simulink model "EnablePort2"  (R2017b)
settings: Solver=FixedStepDiscrete  StartTime=0.0  StopTime=10.0  FixedStep=0.200000  RelTol=1e-3
model workspace (MAT data in the model file):
  input_struct.time = [0; 0.2; 0.4; 0.6; 0.8; 1; 1.2; 1.4; 1.6; 1.8; 2; 2.2; 2.4; 2.6; 2.8; 3; 3.2; 3.4; 3.6; 3.8; 4; 4.2; 4.4; 4.6; 4.8; 5; 5.2; 5.4; 5.6; 5.8; 6; 6.2; 6.4; 6.6; 6.8; 7; 7.2; 7.4; 7.6; 7.8; 8; 8.2; 8.4; 8.6; 8.8; 9; 9.2; 9.4; 9.6; 9.8; 10; 10.2; 10.4; 10.6; 10.8; 11; 11.2; 11.4; 11.6; 11.8; 12; 12.2; 12.4; 12.6; 12.8; 13; 13.2; 13.4; 13.6; 13.8; 14; 14.2; 14.4; 14.6; 14.8; 15; 15.2; 15.4; 15.6; 15.8; 16; 16.2; 16.4; 16.6; 16.8; 17; 17.2; 17.4; 17.6; 17.8; 18; 18.2; 18.4; 18.6; 18.8; 19; 19.2; 19.4; 19.6; 19.8]
  input_struct.signals(1).name = 'In1'
  input_struct.signals(1).values = [57.969273693; 82.7041231105; 6.65087199712; 60.8152888981; 12.5320713222; 50.1752903924; -98.1539291241; -4.64302962846; -49.9340946949; -38.4163483162; 93.3898208851; -58.2391278811; 4.09525055477; -54.8907741205; 13.4395747662; 99.6327052148; -73.6269326538; 90.9353169806; -75.2244977004; -62.7523588484; 29.3005421166; -74.3661845002; -83.7358994286; 31.8454108442; -94.5202297837; 97.0359601658; 7.86618942535; -25.2330166582; 41.3469772282; 89.4822748814; -23.5445302312; 38.5817109897; 20.4142624802; 55.0515424276; 18.3668411358; -24.7640384704; 70.1298399192; -54.8529618431; 59.3916568652; 99.3762012577; -43.7378359258; 42.0761950049; 32.9284134306; -17.0328933637; -0.346019545145; 89.8246051015; 90.63633518; 46.5846623372; -23.0639990752; -91.983454233; 16.5867171862; 12.9425283429; -28.9634765103; 76.0401642003; 24.906026599; 24.803109268; -40.8517177427; -85.0640146214; -41.2588011215; -53.052038291; -30.8205238166; 69.6980718111; -67.927123626; -68.427124744; 1.73185392845; 20.6602000119; -67.7206063001; 27.0908649699; 68.7881151707; 56.4538423892; -47.0867291292; -37.0602075398; -63.3608856957; -10.5053454909; -34.6642766771; -44.0367420079; 86.3527816834; -20.0615174075; -24.1153686312; 18.5692898981; -86.2986628105; -58.9524675794; 44.7236556204; 15.0295225661; -59.9534992726; 68.6960690554; -15.2539997979; 8.95019251945; 5.5934767678; -62.978435841; -83.6620572023; -7.18127540382; -93.8890448599; -13.0031684902; 11.5729922646; 27.7564258613; -93.1565173415; 41.9800894582; -66.1352103091; 18.6764946421]
  input_struct.signals(1).dimensions = 1
  input_struct.signals(2).name = 'Enable'
  input_struct.signals(2).values = [21.6129838653; 54.4719173974; -88.7452768515; 70.9450293897; -23.1431348911; -20.0762077942; -34.9165029203; 11.0780220972; -40.9159793561; -26.7759995931; -30.1903342657; 26.0448111076; 32.8884161614; 98.4192673234; 88.8722524324; -29.9304276267; -61.4004110247; 83.9152276745; -42.2615899335; 10.1718855023; 83.8648307629; -81.9902955723; -48.4607395594; -14.5904084585; 15.5446580081; 79.9042789778; -56.3548766014; 93.4063768947; -13.2037243931; 56.9644846349; 5.0467689241; -33.7446294351; -13.6812706476; 43.5803202039; 83.2424156234; 78.0055974736; -73.0587883246; -76.0174489205; 78.6904842168; 30.6171083505; -91.9443846645; 0.943192710913; 78.8906930826; -22.8543071113; -41.5896244284; -53.1926860055; -59.8103285268; -23.9387873457; 18.9580284497; -46.3228050071; 24.4885283935; 60.9134619765; -79.2057482954; 45.8480614991; 29.7180528831; -5.06907532904; 86.5824220079; -80.7112641316; 19.8213836731; -53.2870581569; -93.5343323586; 15.9718527551; 68.4396304681; 11.3793976245; 67.9765979964; -59.0095452664; 24.2509773626; -65.1958225406; -42.0920362441; -96.2994129362; 40.2992780308; 90.4182743521; 49.8018670091; 51.3454778966; 8.41781508896; -43.5874254242; -51.025030622; -42.7363564351; 92.626882046; -53.860930873; 7.46428268722; -58.9983495565; -13.1917410897; -71.5576055062; -24.8832450068; 58.7121253575; 62.563130171; 80.7581812918; 8.07514683317; 63.5726624463; 41.6833290665; -91.3582296227; -70.8108039161; -53.3328674526; -50.6597837729; -65.943451406; -52.9886329908; -44.9077848095; 90.3213252341; -30.665803355]
  input_struct.signals(2).dimensions = 1
settings Model: Creator=hbourbou  LastModifiedBy=hbourbou
settings DataIOCC: SaveFormat=StructureWithTime
settings OptimizationCC: LifeSpan=inf
settings DebuggingCC: SFExecutionAtInitializationDiag=none
settings HardwareCC: ProdBitPerSizeT=32  ProdBitPerPtrDiffT=32  ProdWordSize=32  ProdHWDeviceType=Specified
settings CodeAppCC: StateflowObjectComments=on

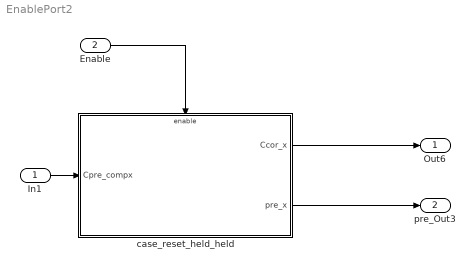
== system EnablePort2 ==
  In1 : Inport
  Enable : Inport  Port=2
  case_reset_held_held : Subsystem  TreatAsAtomicUnit=on
  Out6 : Outport
  pre_Out3 : Outport  Port=2
  wires:
  In1/1 -> case_reset_held_held/1(Cpre_compx)
  case_reset_held_held/1(Ccor_x) -> Out6/1
  case_reset_held_held/2(pre_x) -> pre_Out3/1
  Enable/1 -> case_reset_held_held/Enable

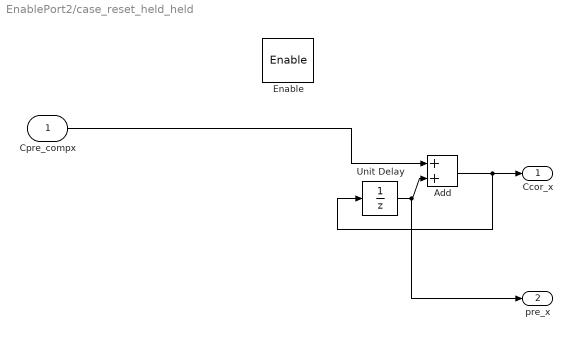
== system EnablePort2/case_reset_held_held ==
  Cpre_compx : Inport  OutDataTypeStr=double  PortDimensions=[1]
  Enable : EnablePort  StatesWhenEnabling=reset
  Add : Sum
  Unit Delay : UnitDelay  SampleTime=-1.0000000000000000
  Ccor_x : Outport  InitialOutput=0
  pre_x : Outport  Port=2  InitialOutput=0
  wires:
  Cpre_compx/1 -> Add/1
  Add/1 -> Unit Delay/1, Ccor_x/1
  Unit Delay/1 -> pre_x/1, Add/2
